simulink model "Unit_Ramp_Response"  (R2021b)
settings: Solver=VariableStepAuto  StartTime=0.0  StopTime=10.0  RelTol=1e-3
libraries: simulink x1
settings Model: Creator=Richi  LastModifiedBy=Richi

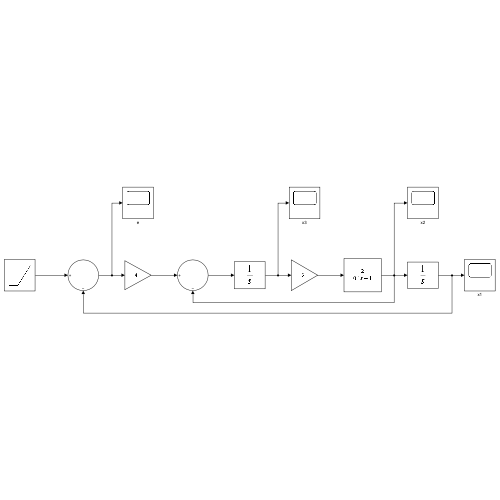
[thumbnail: Simulink's stored preview of the top-level diagram]
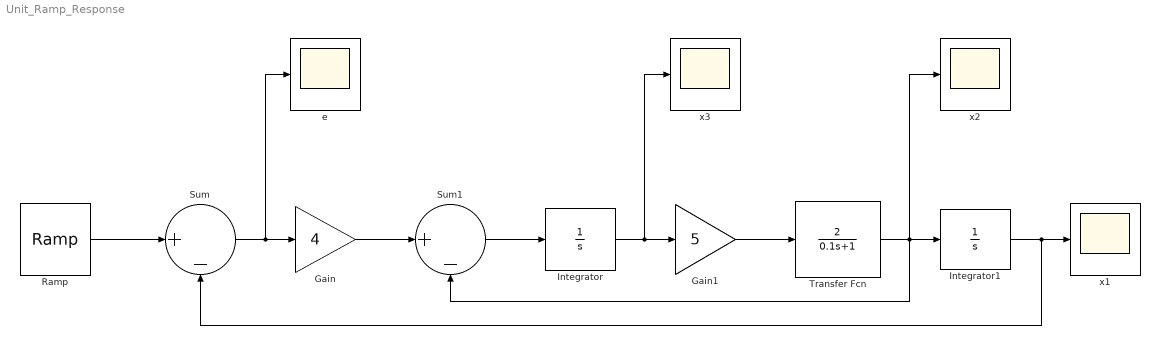
== system Unit_Ramp_Response ==
  Gain : Gain  Gain=4
  Gain1 : Gain  Gain=5
  Integrator : Integrator
  Integrator1 : Integrator
  Ramp : simulink/Sources/Ramp  slope=1  start=0  InitialOutput=0
  Sum : Sum  Inputs=|+-
  Sum1 : Sum  Inputs=|+-
  Transfer Fcn : TransferFcn  Numerator=[2]  Denominator=[0.1 1]
  e : Scope
  x1 : Scope
  x2 : Scope
  x3 : Scope
  wires:
  Sum/1 -> e/1, Gain/1
  Ramp/1 -> Sum/1
  Sum1/1 -> Integrator/1
  Integrator1/1 -> Sum/2, x1/1
  Gain1/1 -> Transfer Fcn/1
  Integrator/1 -> x3/1, Gain1/1
  Gain/1 -> Sum1/1
  Transfer Fcn/1 -> Sum1/2, x2/1, Integrator1/1
